simulink model "SimulationExample3"  (R2016b)
settings: Solver=VariableStepAuto  StartTime=0.0  StopTime=0.3  RelTol=1e-3
libraries: fl_lib x8, nesl_utility x3
settings Model: Creator=mmi-vsa  LastModifiedBy=mmi-vsa

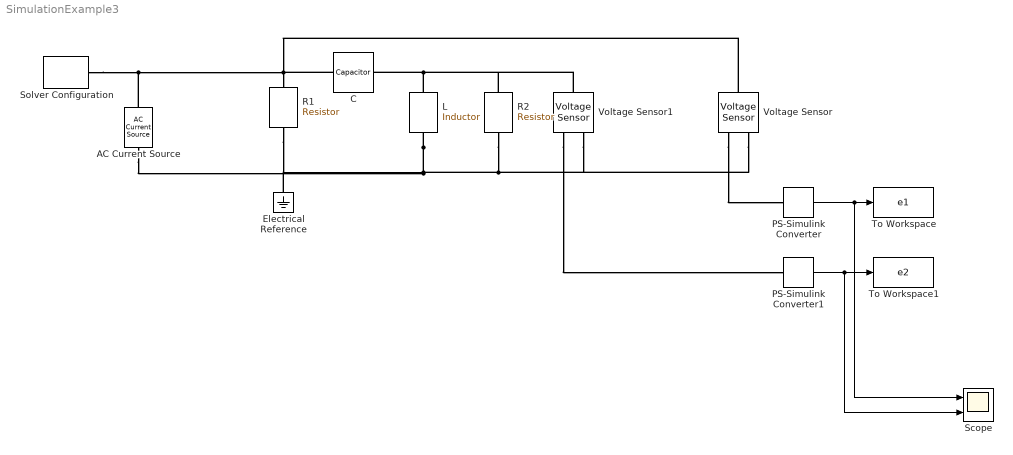
== system SimulationExample3 ==
  AC Current Source : fl_lib/Electrical/Electrical Sources/AC Current Source  amp=10 A  shift=90 deg  frequency=50 Hz  omega=0 rad/s
  C : fl_lib/Electrical/Electrical Elements/Capacitor  c=1 mF  r=0 Ohm  g=0 1/Ohm  i_specify=off  i_priority=None  i=0 A  v_specify=off  v_priority=None  v=0 V  vc_specify=off  vc_priority=High  vc=0 V
  Electrical Reference : fl_lib/Electrical/Electrical Elements/Electrical Reference
  L : fl_lib/Electrical/Electrical Elements/Inductor  l=1 mH  r=0 Ohm  g=0 1/Ohm  i_specify=off  i_priority=None  i=0 A  v_specify=off  v_priority=None  v=0 V  i_L_specify=off  i_L_priority=High  i_L=0 A
  PS-Simulink Converter : nesl_utility/PS-Simulink Converter  PhysicalDomain=network_engine_domain  SubClassName=ps_output  LeftPortType=input  RightPortType=output  PseudoPeriodic=off  Frequencies=[]  Unit=1  AffineConversion=off
  PS-Simulink Converter1 : nesl_utility/PS-Simulink Converter  PhysicalDomain=network_engine_domain  SubClassName=ps_output  LeftPortType=input  RightPortType=output  PseudoPeriodic=off  Frequencies=[]  Unit=1  AffineConversion=off
  R1 : fl_lib/Electrical/Electrical Elements/Resistor  R=1 Ohm  i_specify=off  i_priority=None  i=0 A  v_specify=off  v_priority=None  v=0 V
  R2 : fl_lib/Electrical/Electrical Elements/Resistor  R=1 Ohm  i_specify=off  i_priority=None  i=0 A  v_specify=off  v_priority=None  v=0 V
  Scope : Scope  NumInputPorts=2
  Solver Configuration : nesl_utility/Solver Configuration  PhysicalDomain=network_engine_domain  SubClassName=solver  LeftPortType=input  RightPortType=generic  Accelerate=off  Tones=[]  Harmonics=[]  SimulateNoise=off  Profile=off  UseLocalSampling=off  EnableSwitchedLinearOptims=on  FrequencyDomain=off  UseCCode=off  RelTol=0.001  AbsTol=1e-06  MinStep=1e-09  ToWorkspace=off  RevertToSquareIcSolve=off  NumHomotopyIterations=100  PhasorMode=off  PhasorModeNumHarmonics=1  OverrideAbsTol=off  DoDC=off  ResidualTolerance=1e-09  UseLocalSolver=on  LocalSolverChoice=NE_TRAPEZOIDAL_ADVANCER  LocalSolverSampleTime=0.001  DoFixedCost=on  MaxNonlinIter=3  MaxModeIter=2  LinearAlgebra=Sparse  DelaysMemoryBudget=1024  AutomaticFiltering=on  FilteringTimeConstant=0.001
  To Workspace : ToWorkspace  VariableName=e1  SampleTime=-1
  To Workspace1 : ToWorkspace  VariableName=e2  SampleTime=-1
  Voltage Sensor : fl_lib/Electrical/Electrical Sensors/Voltage Sensor
  Voltage Sensor1 : fl_lib/Electrical/Electrical Sensors/Voltage Sensor
  wires:
  PS-Simulink Converter/1 -> Scope/1, To Workspace/1
  PS-Simulink Converter1/1 -> Scope/2, To Workspace1/1
  connections:
  L/LConn1 -- R2/LConn1 -- Voltage Sensor1/LConn1 -- C/RConn1
  Solver Configuration/RConn1 -- AC Current Source/LConn1 -- Voltage Sensor/LConn1 -- C/LConn1 -- R1/LConn1
  L/RConn1 -- R2/RConn1 -- Voltage Sensor/RConn2 -- Voltage Sensor1/RConn2 -- AC Current Source/RConn1 -- Electrical Reference/LConn1 -- R1/RConn1
  Voltage Sensor/RConn1 -- PS-Simulink Converter/LConn1
  Voltage Sensor1/RConn1 -- PS-Simulink Converter1/LConn1
